simulink model "adc16_dbf_4fft"  (R2013a)
settings: Solver=ode45  StartTime=0.0  StopTime=2050  RelTol=1e-3
undefined symbols (not defined in the file): pfb_coeff_gen_calc
libraries: xbsIndex_r4 x1713, casper_library_misc x294, casper_library_delays x48, casper_library_pfbs x16, simulink x16, xps_library x1
(part 4 of 21)

== system adc16_dbf_4fft/sync_gen ==
  Constant : Constant
  Constant1 : Constant  Value=0
  Constant2 : Constant  Value=0
  Counter3 : xbsIndex_r4/Counter  cnt_type=Free Running  cnt_to=Inf  operation=Up  start_count=0  cnt_by_val=1  arith_type=Unsigned  n_bits=32  bin_pt=0  load_pin=off  rst=on  en=off  explicit_period=off  period=1  dbl_ovrd=off  use_behavioral_HDL=on  implementation=Fabric  use_rpm=on  block_type=counter
      settings: xl_area=[0, 0, 0, 0, 0, 0, 0]
  Logical : xbsIndex_r4/Logical  logical_function=OR  inputs=2  en=off  latency=0  precision=Full  arith_type=Unsigned  n_bits=8  bin_pt=2  align_bp=on  dbl_ovrd=off  block_type=logical
      settings: xl_area=[0, 0, 0, 0, 0, 0, 0]
  Logical1 : xbsIndex_r4/Logical  logical_function=OR  inputs=2  en=off  latency=0  precision=Full  arith_type=Unsigned  n_bits=8  bin_pt=2  align_bp=on  dbl_ovrd=off  block_type=logical
      settings: xl_area=[0, 0, 0, 0, 0, 0, 0]
  Mux : xbsIndex_r4/Mux  inputs=2  en=off  latency=0  precision=Full  arith_type=Unsigned  n_bits=16  bin_pt=14  quantization=Truncate  overflow=Wrap  dbl_ovrd=off  block_type=mux
  Relational : xbsIndex_r4/Relational  mode=a=b  en=off  latency=1  dbl_ovrd=off  block_type=relational
      settings: xl_area=[0, 0, 0, 0, 0, 0, 0]  block_version=10.1.3
  Slice1 : xbsIndex_r4/Slice  nbits=1  boolean_output=on  mode=Lower Bit Location + Width  bit1=0  base1=MSB of Input  bit0=0  base0=LSB of Input  dbl_ovrd=off  block_type=slice
      settings: infoedit="Extracts a given range of bits from each input sample and presents it at the output.  The output type is ordinarily unsigned with binary point at zero, but can be Boolean when the slice is one bit wide.<P><P>Hardware notes: In hardware this block costs nothing."  block_version=10.1.3
  Slice2 : xbsIndex_r4/Slice  nbits=1  boolean_output=on  mode=Lower Bit Location + Width  bit1=0  base1=MSB of Input  bit0=0  base0=LSB of Input  dbl_ovrd=off  block_type=slice
      settings: infoedit="Extracts a given range of bits from each input sample and presents it at the output.  The output type is ordinarily unsigned with binary point at zero, but can be Boolean when the slice is one bit wide.<P><P>Hardware notes: In hardware this block costs nothing."  block_version=10.1.3
  posedge1 : casper_library_misc/edge_detect  edge=Rising  polarity=Active High  x_in=[0 0.08 0.08 0.16 0.16 0.24 0.24 0.32 0.32 0.4]  y_in="[-1 -1  1  1  1  1  1  1  1  1]"  x_out=[0.6 0.68 0.68 0.76 0.76 0.84 0.84 0.92 0.92 1]  y_out="[-1 -1  1  1 -1 -1 -1 -1 -1 -1]"
  posedge3 : casper_library_misc/edge_detect  edge=Rising  polarity=Active High  x_in=[0 0.08 0.08 0.16 0.16 0.24 0.24 0.32 0.32 0.4]  y_in="[-1 -1  1  1  1  1  1  1  1  1]"  x_out=[0.6 0.68 0.68 0.76 0.76 0.84 0.84 0.92 0.92 1]  y_out="[-1 -1  1  1 -1 -1 -1 -1 -1 -1]"
  sync : Subsystem  Tag=xps:sw_reg  AncestorBlock=xps_library/software_register  mask(swreg){mode=one value, io_dir=From Processor, io_delay=0, sample_period=1, names=reg, bitwidths=32, arith_types=0, bin_pts=0, sim_port=on, show_format=off}
      mask prompts: io_dir "I/O direction"; io_delay "I/O delay"; sample_period "Sample period"; names "Name:"; bitwidths "Bitwidth:"; arith_types "Type (ufix=0, fix=1, bool=2):"; bin_pts "Binary pt:"; sim_port "Provide sim input/output?"; show_format "Print format string?"
      mask init:
      | swreg_init(gcb)
      settings: AttributesFormatString=1input
      mask TypeOptions mode: one value | fields of equal size | fields of arbitrary size
      mask Callback mode: swreg_cb(gcb);
      mask TypeOptions io_dir: To Processor | From Processor
      mask Callback io_dir:
      | mask_enables = get_param(gcb, 'MaskEnables');
      | mask_names = get_param(gcb, 'MaskNames');
      | if strcmp(get_param(gcb, 'io_dir'), 'To Processor'),
      |     mask_enables{ismember(mask_names, 'sample_period')} = 'off';
      | else
      |     mask_enables{ismember(mask_names, 'sample_period')} = 'on';
      | end
      | set_param(gcb, 'MaskEnables', mask_enables);
      mask Callback bitwidths:
      | swreg_maskcheck(gcb);
      | % blk = gcb;
      | % mode = get_param(blk, 'mode');
      | % current_widths = eval(get_param(blk, 'bitwidths'));
      | % if (strcmp(mode, 'one value') || strcmp(mode, 'fields of equal size')) && (length(current_widths) > 1),
      | %     error('Only one width may be specified for this mode.');
      | % elseif strcmp(mode, 'fields of arbitrary size')
      | %     current_names = textscan(strtrim(strrep(strrep(get_param(blk, 'names'), ']', ''), '[', '')), '%s');
      | %     current_names = current_names{1};
      | %     numios = length(current_names);
      | %     if length(current_widths) ~= numios,
      | %         error('%d field names specified, but %d widths?', numios, length(current_widths));
      | %     end
      | % end
      | % total_width = 0;
      | % for ctr = 1 : length(current_widths),
      | %     total_width = total_width + current_widths(ctr);
      | % end
      | % if total_width > 32,
      | %     error('Total width must be 32 or less, set to %d.', total_width);
      | % end
      mask Callback arith_types:
      | [numios, ~, ~, ~, current_types] = swreg_maskcheck(gcb);
      | % blk = gcb;
      | % mode = get_param(blk, 'mode');
      | % current_types = eval(get_param(blk, 'arith_types'));
      | % numios = length(current_types);
      | % if (strcmp(mode, 'one value') || strcmp(mode, 'fields of equal size')) && (length(current_types) > 1),
      | %     error('Only one type may be specified for this mode.');
      | % elseif strcmp(mode, 'fields of arbitrary size')
      | %     current_names = textscan(strtrim(strrep(strrep(get_param(blk, 'names'), ']', ''), '[', '')), '%s');
      | %     current_names = current_names{1};
      | %     numios = length(current_names);
      | %     if length(current_types) ~= numios,
      | %         error('%d field names specified, but %d types?', numios, length(current_types));
      | %     end
      | % end
      | problem = 0;
      | for ctr = 1 : numios,
      |     t = current_types(ctr);
      |     if (t < 0) || (t > 2),
      |         problem = t;
      |         ctr = numios + 1;
      |     end
      | end
      | if problem ~= 0,
      |     error('Type cannot be %i, must be 0, 1 or 2.', problem);
      | end
      mask Callback bin_pts:
      | swreg_maskcheck(gcb);
      | % blk = gcb;
      | % mode = get_param(blk, 'mode');
      | % current_bins = eval(get_param(blk, 'bin_pts'));
      | % if (strcmp(mode, 'one value') || strcmp(mode, 'fields of equal size')) && (length(current_bins) > 1),
      | %     error('Only one binary pt may be specified for this mode.');
      | % elseif strcmp(mode, 'fields of arbitrary size')
      | %     current_names = textscan(strtrim(strrep(strrep(get_param(blk, 'names'), ']', ''), '[', '')), '%s');
      | %     current_names = current_names{1};
      | %     numios = length(current_names);
      | %     if length(current_bins) ~= numios,
      | %         error('%d field names specified, but %d binary pts?', numios, length(current_bins));
      | %     end
      | % end
  sync_period_const : xbsIndex_r4/Constant  const=1022  gui_display_data_type=Fixed-point  arith_type=Signed (2's comp)  n_bits=32  bin_pt=0  preci_type=Single  exp_width=8  frac_width=24  explicit_period=off  period=1  equ=P=C  opselect=C  inp2=PCIN>>17  opr=+  inp1=P  carry=CIN  dbl_ovrd=off  block_type=constant
      settings: block_version=10.1.1
  sync_period_sel : Subsystem  Tag=xps:sw_reg  AncestorBlock=xps_library/software_register  mask(swreg){mode=one value, io_dir=From Processor, io_delay=0, sample_period=1, names=reg, bitwidths=32, arith_types=0, bin_pts=0, sim_port=on, show_format=off}
      mask prompts: io_dir "I/O direction"; io_delay "I/O delay"; sample_period "Sample period"; names "Name:"; bitwidths "Bitwidth:"; arith_types "Type (ufix=0, fix=1, bool=2):"; bin_pts "Binary pt:"; sim_port "Provide sim input/output?"; show_format "Print format string?"
      mask init:
      | swreg_init(gcb)
      settings: AttributesFormatString=1input
      mask TypeOptions mode: one value | fields of equal size | fields of arbitrary size
      mask Callback mode: swreg_cb(gcb);
      mask TypeOptions io_dir: To Processor | From Processor
      mask Callback io_dir:
      | mask_enables = get_param(gcb, 'MaskEnables');
      | mask_names = get_param(gcb, 'MaskNames');
      | if strcmp(get_param(gcb, 'io_dir'), 'To Processor'),
      |     mask_enables{ismember(mask_names, 'sample_period')} = 'off';
      | else
      |     mask_enables{ismember(mask_names, 'sample_period')} = 'on';
      | end
      | set_param(gcb, 'MaskEnables', mask_enables);
      mask Callback bitwidths:
      | swreg_maskcheck(gcb);
      | % blk = gcb;
      | % mode = get_param(blk, 'mode');
      | % current_widths = eval(get_param(blk, 'bitwidths'));
      | % if (strcmp(mode, 'one value') || strcmp(mode, 'fields of equal size')) && (length(current_widths) > 1),
      | %     error('Only one width may be specified for this mode.');
      | % elseif strcmp(mode, 'fields of arbitrary size')
      | %     current_names = textscan(strtrim(strrep(strrep(get_param(blk, 'names'), ']', ''), '[', '')), '%s');
      | %     current_names = current_names{1};
      | %     numios = length(current_names);
      | %     if length(current_widths) ~= numios,
      | %         error('%d field names specified, but %d widths?', numios, length(current_widths));
      | %     end
      | % end
      | % total_width = 0;
      | % for ctr = 1 : length(current_widths),
      | %     total_width = total_width + current_widths(ctr);
      | % end
      | % if total_width > 32,
      | %     error('Total width must be 32 or less, set to %d.', total_width);
      | % end
      mask Callback arith_types:
      | [numios, ~, ~, ~, current_types] = swreg_maskcheck(gcb);
      | % blk = gcb;
      | % mode = get_param(blk, 'mode');
      | % current_types = eval(get_param(blk, 'arith_types'));
      | % numios = length(current_types);
      | % if (strcmp(mode, 'one value') || strcmp(mode, 'fields of equal size')) && (length(current_types) > 1),
      | %     error('Only one type may be specified for this mode.');
      | % elseif strcmp(mode, 'fields of arbitrary size')
      | %     current_names = textscan(strtrim(strrep(strrep(get_param(blk, 'names'), ']', ''), '[', '')), '%s');
      | %     current_names = current_names{1};
      | %     numios = length(current_names);
      | %     if length(current_types) ~= numios,
      | %         error('%d field names specified, but %d types?', numios, length(current_types));
      | %     end
      | % end
      | problem = 0;
      | for ctr = 1 : numios,
      |     t = current_types(ctr);
      |     if (t < 0) || (t > 2),
      |         problem = t;
      |         ctr = numios + 1;
      |     end
      | end
      | if problem ~= 0,
      |     error('Type cannot be %i, must be 0, 1 or 2.', problem);
      | end
      mask Callback bin_pts:
      | swreg_maskcheck(gcb);
      | % blk = gcb;
      | % mode = get_param(blk, 'mode');
      | % current_bins = eval(get_param(blk, 'bin_pts'));
      | % if (strcmp(mode, 'one value') || strcmp(mode, 'fields of equal size')) && (length(current_bins) > 1),
      | %     error('Only one binary pt may be specified for this mode.');
      | % elseif strcmp(mode, 'fields of arbitrary size')
      | %     current_names = textscan(strtrim(strrep(strrep(get_param(blk, 'names'), ']', ''), '[', '')), '%s');
      | %     current_names = current_names{1};
      | %     numios = length(current_names);
      | %     if length(current_bins) ~= numios,
      | %         error('%d field names specified, but %d binary pts?', numios, length(current_bins));
      | %     end
      | % end
  sync_period_var : Subsystem  Tag=xps:sw_reg  AncestorBlock=xps_library/software_register  mask(swreg){mode=one value, io_dir=From Processor, io_delay=0, sample_period=1, names=reg, bitwidths=32, arith_types=0, bin_pts=0, sim_port=on, show_format=off}
      mask prompts: io_dir "I/O direction"; io_delay "I/O delay"; sample_period "Sample period"; names "Name:"; bitwidths "Bitwidth:"; arith_types "Type (ufix=0, fix=1, bool=2):"; bin_pts "Binary pt:"; sim_port "Provide sim input/output?"; show_format "Print format string?"
      mask init:
      | swreg_init(gcb)
      settings: AttributesFormatString=1input
      mask TypeOptions mode: one value | fields of equal size | fields of arbitrary size
      mask Callback mode: swreg_cb(gcb);
      mask TypeOptions io_dir: To Processor | From Processor
      mask Callback io_dir:
      | mask_enables = get_param(gcb, 'MaskEnables');
      | mask_names = get_param(gcb, 'MaskNames');
      | if strcmp(get_param(gcb, 'io_dir'), 'To Processor'),
      |     mask_enables{ismember(mask_names, 'sample_period')} = 'off';
      | else
      |     mask_enables{ismember(mask_names, 'sample_period')} = 'on';
      | end
      | set_param(gcb, 'MaskEnables', mask_enables);
      mask Callback bitwidths:
      | swreg_maskcheck(gcb);
      | % blk = gcb;
      | % mode = get_param(blk, 'mode');
      | % current_widths = eval(get_param(blk, 'bitwidths'));
      | % if (strcmp(mode, 'one value') || strcmp(mode, 'fields of equal size')) && (length(current_widths) > 1),
      | %     error('Only one width may be specified for this mode.');
      | % elseif strcmp(mode, 'fields of arbitrary size')
      | %     current_names = textscan(strtrim(strrep(strrep(get_param(blk, 'names'), ']', ''), '[', '')), '%s');
      | %     current_names = current_names{1};
      | %     numios = length(current_names);
      | %     if length(current_widths) ~= numios,
      | %         error('%d field names specified, but %d widths?', numios, length(current_widths));
      | %     end
      | % end
      | % total_width = 0;
      | % for ctr = 1 : length(current_widths),
      | %     total_width = total_width + current_widths(ctr);
      | % end
      | % if total_width > 32,
      | %     error('Total width must be 32 or less, set to %d.', total_width);
      | % end
      mask Callback arith_types:
      | [numios, ~, ~, ~, current_types] = swreg_maskcheck(gcb);
      | % blk = gcb;
      | % mode = get_param(blk, 'mode');
      | % current_types = eval(get_param(blk, 'arith_types'));
      | % numios = length(current_types);
      | % if (strcmp(mode, 'one value') || strcmp(mode, 'fields of equal size')) && (length(current_types) > 1),
      | %     error('Only one type may be specified for this mode.');
      | % elseif strcmp(mode, 'fields of arbitrary size')
      | %     current_names = textscan(strtrim(strrep(strrep(get_param(blk, 'names'), ']', ''), '[', '')), '%s');
      | %     current_names = current_names{1};
      | %     numios = length(current_names);
      | %     if length(current_types) ~= numios,
      | %         error('%d field names specified, but %d types?', numios, length(current_types));
      | %     end
      | % end
      | problem = 0;
      | for ctr = 1 : numios,
      |     t = current_types(ctr);
      |     if (t < 0) || (t > 2),
      |         problem = t;
      |         ctr = numios + 1;
      |     end
      | end
      | if problem ~= 0,
      |     error('Type cannot be %i, must be 0, 1 or 2.', problem);
      | end
      mask Callback bin_pts:
      | swreg_maskcheck(gcb);
      | % blk = gcb;
      | % mode = get_param(blk, 'mode');
      | % current_bins = eval(get_param(blk, 'bin_pts'));
      | % if (strcmp(mode, 'one value') || strcmp(mode, 'fields of equal size')) && (length(current_bins) > 1),
      | %     error('Only one binary pt may be specified for this mode.');
      | % elseif strcmp(mode, 'fields of arbitrary size')
      | %     current_names = textscan(strtrim(strrep(strrep(get_param(blk, 'names'), ']', ''), '[', '')), '%s');
      | %     current_names = current_names{1};
      | %     numios = length(current_names);
      | %     if length(current_bins) ~= numios,
      | %         error('%d field names specified, but %d binary pts?', numios, length(current_bins));
      | %     end
      | % end
  sync_out : Outport
  wires:
  Constant2/1 -> sync_period_var/1(sim_1)
  sync_period_var/1(in_reg) -> Mux/3
  sync_period_const/1 -> Mux/2
  Slice1/1 -> Mux/1
  sync_period_sel/1(in_reg) -> Slice1/1
  Constant1/1 -> sync_period_sel/1(sim_1)
  Mux/1 -> Relational/1
  posedge1/1 -> sync_out/1
  Logical/1 -> posedge1/1
  Relational/1 -> Logical1/1, Logical/1
  Counter3/1 -> Relational/2
  Logical1/1 -> Counter3/1
  Slice2/1 -> Logical/2, Logical1/2
  posedge3/1 -> Slice2/1
  sync/1(in_reg) -> posedge3/1
  Constant/1 -> sync/1(sim_1)

== system adc16_dbf_4fft/4fft/mult_j ==
  a+jb : Inport
  Negate : xbsIndex_r4/Negate  precision=User Defined  arith_type="Signed  (2's comp)"  n_bits=18  bin_pt=17  quantization=Truncate  overflow=Wrap  en=off  latency=0  dbl_ovrd=off  block_type=negate
  c_to_ri : casper_library_misc/c_to_ri  n_bits=18  bin_pt=17
  ri_to_c : casper_library_misc/ri_to_c
  ja-b : Outport
  wires:
  a+jb/1 -> c_to_ri/1
  ri_to_c/1 -> ja-b/1
  c_to_ri/2 -> Negate/1
  c_to_ri/1 -> ri_to_c/2
  Negate/1 -> ri_to_c/1

== system adc16_dbf_4fft/4fft/mult_jjj ==
  a+jb : Inport
  Negate : xbsIndex_r4/Negate  precision=User Defined  arith_type="Signed  (2's comp)"  n_bits=18  bin_pt=17  quantization=Truncate  overflow=Wrap  en=off  latency=0  dbl_ovrd=off  block_type=negate
  c_to_ri : casper_library_misc/c_to_ri  n_bits=18  bin_pt=17
  ri_to_c : casper_library_misc/ri_to_c
  b-ja : Outport
  wires:
  ri_to_c/1 -> b-ja/1
  a+jb/1 -> c_to_ri/1
  c_to_ri/2 -> ri_to_c/1
  c_to_ri/1 -> Negate/1
  Negate/1 -> ri_to_c/2

== system adc16_dbf_4fft/4fft/pipeline ==
  d : Inport
  Register{0..3} (4 alike) : xbsIndex_r4/Register  init=0  rst=off  en=off  dbl_ovrd=off  block_type=register
      Register0 settings: block_version=11.4
      Register1 settings: block_version=11.4
  q : Outport
  wires:
  Register0/1 -> Register1/1
  Register1/1 -> Register2/1
  Register2/1 -> Register3/1
  d/1 -> Register0/1
  Register3/1 -> q/1

== system adc16_dbf_4fft/4fft/pipeline1 ==
  d : Inport
  Register{0..3} (4 alike) : xbsIndex_r4/Register  init=0  rst=off  en=off  dbl_ovrd=off  block_type=register
      Register0 settings: block_version=11.4
      Register1 settings: block_version=11.4
  q : Outport
  wires:
  Register0/1 -> Register1/1
  Register1/1 -> Register2/1
  Register2/1 -> Register3/1
  d/1 -> Register0/1
  Register3/1 -> q/1

== system adc16_dbf_4fft/4fft/real2complex ==
  r : Inport
  c_to_ri : casper_library_misc/c_to_ri  n_bits=18  bin_pt=17
  ri_to_c : casper_library_misc/ri_to_c
  c : Outport
  wires:
  c_to_ri/2 -> ri_to_c/2
  r/1 -> c_to_ri/1
  c_to_ri/1 -> ri_to_c/1
  ri_to_c/1 -> c/1

== system adc16_dbf_4fft/4fft/real2complex1 ==
  r : Inport
  c_to_ri : casper_library_misc/c_to_ri  n_bits=18  bin_pt=17
  ri_to_c : casper_library_misc/ri_to_c
  c : Outport
  wires:
  ri_to_c/1 -> c/1
  c_to_ri/1 -> ri_to_c/1
  r/1 -> c_to_ri/1
  c_to_ri/2 -> ri_to_c/2

== system adc16_dbf_4fft/4fft/real2complex2 ==
  r : Inport
  c_to_ri : casper_library_misc/c_to_ri  n_bits=18  bin_pt=17
  ri_to_c : casper_library_misc/ri_to_c
  c : Outport
  wires:
  c_to_ri/2 -> ri_to_c/2
  r/1 -> c_to_ri/1
  c_to_ri/1 -> ri_to_c/1
  ri_to_c/1 -> c/1

== system adc16_dbf_4fft/4fft/real2complex3 ==
  r : Inport
  c_to_ri : casper_library_misc/c_to_ri  n_bits=18  bin_pt=17
  ri_to_c : casper_library_misc/ri_to_c
  c : Outport
  wires:
  ri_to_c/1 -> c/1
  c_to_ri/1 -> ri_to_c/1
  r/1 -> c_to_ri/1
  c_to_ri/2 -> ri_to_c/2

== system adc16_dbf_4fft/4fft1/mult_j ==
  a+jb : Inport
  Negate : xbsIndex_r4/Negate  precision=User Defined  arith_type="Signed  (2's comp)"  n_bits=18  bin_pt=17  quantization=Truncate  overflow=Wrap  en=off  latency=0  dbl_ovrd=off  block_type=negate
  c_to_ri : casper_library_misc/c_to_ri  n_bits=18  bin_pt=17
  ri_to_c : casper_library_misc/ri_to_c
  ja-b : Outport
  wires:
  Negate/1 -> ri_to_c/1
  c_to_ri/1 -> ri_to_c/2
  c_to_ri/2 -> Negate/1
  ri_to_c/1 -> ja-b/1
  a+jb/1 -> c_to_ri/1

== system adc16_dbf_4fft/4fft1/mult_jjj ==
  a+jb : Inport
  Negate : xbsIndex_r4/Negate  precision=User Defined  arith_type="Signed  (2's comp)"  n_bits=18  bin_pt=17  quantization=Truncate  overflow=Wrap  en=off  latency=0  dbl_ovrd=off  block_type=negate
  c_to_ri : casper_library_misc/c_to_ri  n_bits=18  bin_pt=17
  ri_to_c : casper_library_misc/ri_to_c
  b-ja : Outport
  wires:
  Negate/1 -> ri_to_c/2
  c_to_ri/1 -> Negate/1
  c_to_ri/2 -> ri_to_c/1
  a+jb/1 -> c_to_ri/1
  ri_to_c/1 -> b-ja/1

== system adc16_dbf_4fft/4fft1/pipeline ==
  d : Inport
  Register{0..3} (4 alike) : xbsIndex_r4/Register  init=0  rst=off  en=off  dbl_ovrd=off  block_type=register
      Register0 settings: block_version=11.4
      Register1 settings: block_version=11.4
  q : Outport
  wires:
  Register3/1 -> q/1
  d/1 -> Register0/1
  Register2/1 -> Register3/1
  Register1/1 -> Register2/1
  Register0/1 -> Register1/1

== system adc16_dbf_4fft/4fft1/pipeline1 ==
  d : Inport
  Register{0..3} (4 alike) : xbsIndex_r4/Register  init=0  rst=off  en=off  dbl_ovrd=off  block_type=register
      Register0 settings: block_version=11.4
      Register1 settings: block_version=11.4
  q : Outport
  wires:
  Register3/1 -> q/1
  d/1 -> Register0/1
  Register2/1 -> Register3/1
  Register1/1 -> Register2/1
  Register0/1 -> Register1/1

== system adc16_dbf_4fft/4fft1/real2complex ==
  r : Inport
  c_to_ri : casper_library_misc/c_to_ri  n_bits=18  bin_pt=17
  ri_to_c : casper_library_misc/ri_to_c
  c : Outport
  wires:
  ri_to_c/1 -> c/1
  c_to_ri/1 -> ri_to_c/1
  r/1 -> c_to_ri/1
  c_to_ri/2 -> ri_to_c/2

== system adc16_dbf_4fft/4fft1/real2complex1 ==
  r : Inport
  c_to_ri : casper_library_misc/c_to_ri  n_bits=18  bin_pt=17
  ri_to_c : casper_library_misc/ri_to_c
  c : Outport
  wires:
  c_to_ri/2 -> ri_to_c/2
  r/1 -> c_to_ri/1
  c_to_ri/1 -> ri_to_c/1
  ri_to_c/1 -> c/1

== system adc16_dbf_4fft/4fft1/real2complex2 ==
  r : Inport
  c_to_ri : casper_library_misc/c_to_ri  n_bits=18  bin_pt=17
  ri_to_c : casper_library_misc/ri_to_c
  c : Outport
  wires:
  ri_to_c/1 -> c/1
  c_to_ri/1 -> ri_to_c/1
  r/1 -> c_to_ri/1
  c_to_ri/2 -> ri_to_c/2

== system adc16_dbf_4fft/4fft1/real2complex3 ==
  r : Inport
  c_to_ri : casper_library_misc/c_to_ri  n_bits=18  bin_pt=17
  ri_to_c : casper_library_misc/ri_to_c
  c : Outport
  wires:
  c_to_ri/2 -> ri_to_c/2
  r/1 -> c_to_ri/1
  c_to_ri/1 -> ri_to_c/1
  ri_to_c/1 -> c/1

== system adc16_dbf_4fft/4fft2/mult_j ==
  a+jb : Inport
  Negate : xbsIndex_r4/Negate  precision=User Defined  arith_type="Signed  (2's comp)"  n_bits=18  bin_pt=17  quantization=Truncate  overflow=Wrap  en=off  latency=0  dbl_ovrd=off  block_type=negate
  c_to_ri : casper_library_misc/c_to_ri  n_bits=18  bin_pt=17
  ri_to_c : casper_library_misc/ri_to_c
  ja-b : Outport
  wires:
  a+jb/1 -> c_to_ri/1
  ri_to_c/1 -> ja-b/1
  c_to_ri/2 -> Negate/1
  c_to_ri/1 -> ri_to_c/2
  Negate/1 -> ri_to_c/1

== system adc16_dbf_4fft/4fft2/mult_jjj ==
  a+jb : Inport
  Negate : xbsIndex_r4/Negate  precision=User Defined  arith_type="Signed  (2's comp)"  n_bits=18  bin_pt=17  quantization=Truncate  overflow=Wrap  en=off  latency=0  dbl_ovrd=off  block_type=negate
  c_to_ri : casper_library_misc/c_to_ri  n_bits=18  bin_pt=17
  ri_to_c : casper_library_misc/ri_to_c
  b-ja : Outport
  wires:
  ri_to_c/1 -> b-ja/1
  a+jb/1 -> c_to_ri/1
  c_to_ri/2 -> ri_to_c/1
  c_to_ri/1 -> Negate/1
  Negate/1 -> ri_to_c/2

== system adc16_dbf_4fft/4fft2/pipeline ==
  d : Inport
  Register{0..3} (4 alike) : xbsIndex_r4/Register  init=0  rst=off  en=off  dbl_ovrd=off  block_type=register
      Register0 settings: block_version=11.4
      Register1 settings: block_version=11.4
  q : Outport
  wires:
  Register0/1 -> Register1/1
  Register1/1 -> Register2/1
  Register2/1 -> Register3/1
  d/1 -> Register0/1
  Register3/1 -> q/1

== system adc16_dbf_4fft/4fft2/pipeline1 ==
  d : Inport
  Register{0..3} (4 alike) : xbsIndex_r4/Register  init=0  rst=off  en=off  dbl_ovrd=off  block_type=register
      Register0 settings: block_version=11.4
      Register1 settings: block_version=11.4
  q : Outport
  wires:
  Register0/1 -> Register1/1
  Register1/1 -> Register2/1
  Register2/1 -> Register3/1
  d/1 -> Register0/1
  Register3/1 -> q/1

== system adc16_dbf_4fft/4fft2/real2complex ==
  r : Inport
  c_to_ri : casper_library_misc/c_to_ri  n_bits=18  bin_pt=17
  ri_to_c : casper_library_misc/ri_to_c
  c : Outport
  wires:
  c_to_ri/2 -> ri_to_c/2
  r/1 -> c_to_ri/1
  c_to_ri/1 -> ri_to_c/1
  ri_to_c/1 -> c/1

== system adc16_dbf_4fft/4fft2/real2complex1 ==
  r : Inport
  c_to_ri : casper_library_misc/c_to_ri  n_bits=18  bin_pt=17
  ri_to_c : casper_library_misc/ri_to_c
  c : Outport
  wires:
  ri_to_c/1 -> c/1
  c_to_ri/1 -> ri_to_c/1
  r/1 -> c_to_ri/1
  c_to_ri/2 -> ri_to_c/2

== system adc16_dbf_4fft/4fft2/real2complex2 ==
  r : Inport
  c_to_ri : casper_library_misc/c_to_ri  n_bits=18  bin_pt=17
  ri_to_c : casper_library_misc/ri_to_c
  c : Outport
  wires:
  c_to_ri/2 -> ri_to_c/2
  r/1 -> c_to_ri/1
  c_to_ri/1 -> ri_to_c/1
  ri_to_c/1 -> c/1

== system adc16_dbf_4fft/4fft2/real2complex3 ==
  r : Inport
  c_to_ri : casper_library_misc/c_to_ri  n_bits=18  bin_pt=17
  ri_to_c : casper_library_misc/ri_to_c
  c : Outport
  wires:
  ri_to_c/1 -> c/1
  c_to_ri/1 -> ri_to_c/1
  r/1 -> c_to_ri/1
  c_to_ri/2 -> ri_to_c/2

== system adc16_dbf_4fft/4fft3/mult_j ==
  a+jb : Inport
  Negate : xbsIndex_r4/Negate  precision=User Defined  arith_type="Signed  (2's comp)"  n_bits=18  bin_pt=17  quantization=Truncate  overflow=Wrap  en=off  latency=0  dbl_ovrd=off  block_type=negate
  c_to_ri : casper_library_misc/c_to_ri  n_bits=18  bin_pt=17
  ri_to_c : casper_library_misc/ri_to_c
  ja-b : Outport
  wires:
  Negate/1 -> ri_to_c/1
  c_to_ri/1 -> ri_to_c/2
  c_to_ri/2 -> Negate/1
  ri_to_c/1 -> ja-b/1
  a+jb/1 -> c_to_ri/1

== system adc16_dbf_4fft/4fft3/mult_jjj ==
  a+jb : Inport
  Negate : xbsIndex_r4/Negate  precision=User Defined  arith_type="Signed  (2's comp)"  n_bits=18  bin_pt=17  quantization=Truncate  overflow=Wrap  en=off  latency=0  dbl_ovrd=off  block_type=negate
  c_to_ri : casper_library_misc/c_to_ri  n_bits=18  bin_pt=17
  ri_to_c : casper_library_misc/ri_to_c
  b-ja : Outport
  wires:
  Negate/1 -> ri_to_c/2
  c_to_ri/1 -> Negate/1
  c_to_ri/2 -> ri_to_c/1
  a+jb/1 -> c_to_ri/1
  ri_to_c/1 -> b-ja/1

== system adc16_dbf_4fft/4fft3/pipeline ==
  d : Inport
  Register{0..3} (4 alike) : xbsIndex_r4/Register  init=0  rst=off  en=off  dbl_ovrd=off  block_type=register
      Register0 settings: block_version=11.4
      Register1 settings: block_version=11.4
  q : Outport
  wires:
  Register3/1 -> q/1
  d/1 -> Register0/1
  Register2/1 -> Register3/1
  Register1/1 -> Register2/1
  Register0/1 -> Register1/1

== system adc16_dbf_4fft/4fft3/pipeline1 ==
  d : Inport
  Register{0..3} (4 alike) : xbsIndex_r4/Register  init=0  rst=off  en=off  dbl_ovrd=off  block_type=register
      Register0 settings: block_version=11.4
      Register1 settings: block_version=11.4
  q : Outport
  wires:
  Register3/1 -> q/1
  d/1 -> Register0/1
  Register2/1 -> Register3/1
  Register1/1 -> Register2/1
  Register0/1 -> Register1/1

== system adc16_dbf_4fft/4fft3/real2complex ==
  r : Inport
  c_to_ri : casper_library_misc/c_to_ri  n_bits=18  bin_pt=17
  ri_to_c : casper_library_misc/ri_to_c
  c : Outport
  wires:
  ri_to_c/1 -> c/1
  c_to_ri/1 -> ri_to_c/1
  r/1 -> c_to_ri/1
  c_to_ri/2 -> ri_to_c/2

== system adc16_dbf_4fft/4fft3/real2complex1 ==
  r : Inport
  c_to_ri : casper_library_misc/c_to_ri  n_bits=18  bin_pt=17
  ri_to_c : casper_library_misc/ri_to_c
  c : Outport
  wires:
  c_to_ri/2 -> ri_to_c/2
  r/1 -> c_to_ri/1
  c_to_ri/1 -> ri_to_c/1
  ri_to_c/1 -> c/1

== system adc16_dbf_4fft/4fft3/real2complex2 ==
  r : Inport
  c_to_ri : casper_library_misc/c_to_ri  n_bits=18  bin_pt=17
  ri_to_c : casper_library_misc/ri_to_c
  c : Outport
  wires:
  ri_to_c/1 -> c/1
  c_to_ri/1 -> ri_to_c/1
  r/1 -> c_to_ri/1
  c_to_ri/2 -> ri_to_c/2

== system adc16_dbf_4fft/4fft3/real2complex3 ==
  r : Inport
  c_to_ri : casper_library_misc/c_to_ri  n_bits=18  bin_pt=17
  ri_to_c : casper_library_misc/ri_to_c
  c : Outport
  wires:
  c_to_ri/2 -> ri_to_c/2
  r/1 -> c_to_ri/1
  c_to_ri/1 -> ri_to_c/1
  ri_to_c/1 -> c/1

== system adc16_dbf_4fft/4fft4/mult_j ==
  a+jb : Inport
  Negate : xbsIndex_r4/Negate  precision=User Defined  arith_type="Signed  (2's comp)"  n_bits=18  bin_pt=17  quantization=Truncate  overflow=Wrap  en=off  latency=0  dbl_ovrd=off  block_type=negate
  c_to_ri : casper_library_misc/c_to_ri  n_bits=18  bin_pt=17
  ri_to_c : casper_library_misc/ri_to_c
  ja-b : Outport
  wires:
  a+jb/1 -> c_to_ri/1
  ri_to_c/1 -> ja-b/1
  c_to_ri/2 -> Negate/1
  c_to_ri/1 -> ri_to_c/2
  Negate/1 -> ri_to_c/1

== system adc16_dbf_4fft/4fft4/mult_jjj ==
  a+jb : Inport
  Negate : xbsIndex_r4/Negate  precision=User Defined  arith_type="Signed  (2's comp)"  n_bits=18  bin_pt=17  quantization=Truncate  overflow=Wrap  en=off  latency=0  dbl_ovrd=off  block_type=negate
  c_to_ri : casper_library_misc/c_to_ri  n_bits=18  bin_pt=17
  ri_to_c : casper_library_misc/ri_to_c
  b-ja : Outport
  wires:
  ri_to_c/1 -> b-ja/1
  a+jb/1 -> c_to_ri/1
  c_to_ri/2 -> ri_to_c/1
  c_to_ri/1 -> Negate/1
  Negate/1 -> ri_to_c/2

== system adc16_dbf_4fft/4fft4/pipeline ==
  d : Inport
  Register{0..3} (4 alike) : xbsIndex_r4/Register  init=0  rst=off  en=off  dbl_ovrd=off  block_type=register
      Register0 settings: block_version=11.4
      Register1 settings: block_version=11.4
  q : Outport
  wires:
  Register0/1 -> Register1/1
  Register1/1 -> Register2/1
  Register2/1 -> Register3/1
  d/1 -> Register0/1
  Register3/1 -> q/1

== system adc16_dbf_4fft/4fft4/pipeline1 ==
  d : Inport
  Register{0..3} (4 alike) : xbsIndex_r4/Register  init=0  rst=off  en=off  dbl_ovrd=off  block_type=register
      Register0 settings: block_version=11.4
      Register1 settings: block_version=11.4
  q : Outport
  wires:
  Register0/1 -> Register1/1
  Register1/1 -> Register2/1
  Register2/1 -> Register3/1
  d/1 -> Register0/1
  Register3/1 -> q/1

== system adc16_dbf_4fft/4fft4/real2complex ==
  r : Inport
  c_to_ri : casper_library_misc/c_to_ri  n_bits=18  bin_pt=17
  ri_to_c : casper_library_misc/ri_to_c
  c : Outport
  wires:
  c_to_ri/2 -> ri_to_c/2
  r/1 -> c_to_ri/1
  c_to_ri/1 -> ri_to_c/1
  ri_to_c/1 -> c/1

== system adc16_dbf_4fft/4fft4/real2complex1 ==
  r : Inport
  c_to_ri : casper_library_misc/c_to_ri  n_bits=18  bin_pt=17
  ri_to_c : casper_library_misc/ri_to_c
  c : Outport
  wires:
  ri_to_c/1 -> c/1
  c_to_ri/1 -> ri_to_c/1
  r/1 -> c_to_ri/1
  c_to_ri/2 -> ri_to_c/2

== system adc16_dbf_4fft/4fft4/real2complex2 ==
  r : Inport
  c_to_ri : casper_library_misc/c_to_ri  n_bits=18  bin_pt=17
  ri_to_c : casper_library_misc/ri_to_c
  c : Outport
  wires:
  c_to_ri/2 -> ri_to_c/2
  r/1 -> c_to_ri/1
  c_to_ri/1 -> ri_to_c/1
  ri_to_c/1 -> c/1

== system adc16_dbf_4fft/4fft4/real2complex3 ==
  r : Inport
  c_to_ri : casper_library_misc/c_to_ri  n_bits=18  bin_pt=17
  ri_to_c : casper_library_misc/ri_to_c
  c : Outport
  wires:
  ri_to_c/1 -> c/1
  c_to_ri/1 -> ri_to_c/1
  r/1 -> c_to_ri/1
  c_to_ri/2 -> ri_to_c/2

== system adc16_dbf_4fft/4fft5/mult_j ==
  a+jb : Inport
  Negate : xbsIndex_r4/Negate  precision=User Defined  arith_type="Signed  (2's comp)"  n_bits=18  bin_pt=17  quantization=Truncate  overflow=Wrap  en=off  latency=0  dbl_ovrd=off  block_type=negate
  c_to_ri : casper_library_misc/c_to_ri  n_bits=18  bin_pt=17
  ri_to_c : casper_library_misc/ri_to_c
  ja-b : Outport
  wires:
  Negate/1 -> ri_to_c/1
  c_to_ri/1 -> ri_to_c/2
  c_to_ri/2 -> Negate/1
  ri_to_c/1 -> ja-b/1
  a+jb/1 -> c_to_ri/1

== system adc16_dbf_4fft/4fft5/mult_jjj ==
  a+jb : Inport
  Negate : xbsIndex_r4/Negate  precision=User Defined  arith_type="Signed  (2's comp)"  n_bits=18  bin_pt=17  quantization=Truncate  overflow=Wrap  en=off  latency=0  dbl_ovrd=off  block_type=negate
  c_to_ri : casper_library_misc/c_to_ri  n_bits=18  bin_pt=17
  ri_to_c : casper_library_misc/ri_to_c
  b-ja : Outport
  wires:
  Negate/1 -> ri_to_c/2
  c_to_ri/1 -> Negate/1
  c_to_ri/2 -> ri_to_c/1
  a+jb/1 -> c_to_ri/1
  ri_to_c/1 -> b-ja/1

== system adc16_dbf_4fft/4fft5/pipeline ==
  d : Inport
  Register{0..3} (4 alike) : xbsIndex_r4/Register  init=0  rst=off  en=off  dbl_ovrd=off  block_type=register
      Register0 settings: block_version=11.4
      Register1 settings: block_version=11.4
  q : Outport
  wires:
  Register3/1 -> q/1
  d/1 -> Register0/1
  Register2/1 -> Register3/1
  Register1/1 -> Register2/1
  Register0/1 -> Register1/1

== system adc16_dbf_4fft/4fft5/pipeline1 ==
  d : Inport
  Register{0..3} (4 alike) : xbsIndex_r4/Register  init=0  rst=off  en=off  dbl_ovrd=off  block_type=register
      Register0 settings: block_version=11.4
      Register1 settings: block_version=11.4
  q : Outport
  wires:
  Register3/1 -> q/1
  d/1 -> Register0/1
  Register2/1 -> Register3/1
  Register1/1 -> Register2/1
  Register0/1 -> Register1/1

== system adc16_dbf_4fft/4fft5/real2complex ==
  r : Inport
  c_to_ri : casper_library_misc/c_to_ri  n_bits=18  bin_pt=17
  ri_to_c : casper_library_misc/ri_to_c
  c : Outport
  wires:
  ri_to_c/1 -> c/1
  c_to_ri/1 -> ri_to_c/1
  r/1 -> c_to_ri/1
  c_to_ri/2 -> ri_to_c/2

== system adc16_dbf_4fft/4fft5/real2complex1 ==
  r : Inport
  c_to_ri : casper_library_misc/c_to_ri  n_bits=18  bin_pt=17
  ri_to_c : casper_library_misc/ri_to_c
  c : Outport
  wires:
  c_to_ri/2 -> ri_to_c/2
  r/1 -> c_to_ri/1
  c_to_ri/1 -> ri_to_c/1
  ri_to_c/1 -> c/1

== system adc16_dbf_4fft/4fft5/real2complex2 ==
  r : Inport
  c_to_ri : casper_library_misc/c_to_ri  n_bits=18  bin_pt=17
  ri_to_c : casper_library_misc/ri_to_c
  c : Outport
  wires:
  ri_to_c/1 -> c/1
  c_to_ri/1 -> ri_to_c/1
  r/1 -> c_to_ri/1
  c_to_ri/2 -> ri_to_c/2

== system adc16_dbf_4fft/4fft5/real2complex3 ==
  r : Inport
  c_to_ri : casper_library_misc/c_to_ri  n_bits=18  bin_pt=17
  ri_to_c : casper_library_misc/ri_to_c
  c : Outport
  wires:
  c_to_ri/2 -> ri_to_c/2
  r/1 -> c_to_ri/1
  c_to_ri/1 -> ri_to_c/1
  ri_to_c/1 -> c/1

== system adc16_dbf_4fft/4fft6/mult_j ==
  a+jb : Inport
  Negate : xbsIndex_r4/Negate  precision=User Defined  arith_type="Signed  (2's comp)"  n_bits=18  bin_pt=17  quantization=Truncate  overflow=Wrap  en=off  latency=0  dbl_ovrd=off  block_type=negate
  c_to_ri : casper_library_misc/c_to_ri  n_bits=18  bin_pt=17
  ri_to_c : casper_library_misc/ri_to_c
  ja-b : Outport
  wires:
  a+jb/1 -> c_to_ri/1
  ri_to_c/1 -> ja-b/1
  c_to_ri/2 -> Negate/1
  c_to_ri/1 -> ri_to_c/2
  Negate/1 -> ri_to_c/1

== system adc16_dbf_4fft/4fft6/mult_jjj ==
  a+jb : Inport
  Negate : xbsIndex_r4/Negate  precision=User Defined  arith_type="Signed  (2's comp)"  n_bits=18  bin_pt=17  quantization=Truncate  overflow=Wrap  en=off  latency=0  dbl_ovrd=off  block_type=negate
  c_to_ri : casper_library_misc/c_to_ri  n_bits=18  bin_pt=17
  ri_to_c : casper_library_misc/ri_to_c
  b-ja : Outport
  wires:
  ri_to_c/1 -> b-ja/1
  a+jb/1 -> c_to_ri/1
  c_to_ri/2 -> ri_to_c/1
  c_to_ri/1 -> Negate/1
  Negate/1 -> ri_to_c/2

== system adc16_dbf_4fft/4fft6/pipeline ==
  d : Inport
  Register{0..3} (4 alike) : xbsIndex_r4/Register  init=0  rst=off  en=off  dbl_ovrd=off  block_type=register
      Register0 settings: block_version=11.4
      Register1 settings: block_version=11.4
  q : Outport
  wires:
  Register0/1 -> Register1/1
  Register1/1 -> Register2/1
  Register2/1 -> Register3/1
  d/1 -> Register0/1
  Register3/1 -> q/1

== system adc16_dbf_4fft/4fft6/pipeline1 ==
  d : Inport
  Register{0..3} (4 alike) : xbsIndex_r4/Register  init=0  rst=off  en=off  dbl_ovrd=off  block_type=register
      Register0 settings: block_version=11.4
      Register1 settings: block_version=11.4
  q : Outport
  wires:
  Register0/1 -> Register1/1
  Register1/1 -> Register2/1
  Register2/1 -> Register3/1
  d/1 -> Register0/1
  Register3/1 -> q/1

== system adc16_dbf_4fft/4fft6/real2complex ==
  r : Inport
  c_to_ri : casper_library_misc/c_to_ri  n_bits=18  bin_pt=17
  ri_to_c : casper_library_misc/ri_to_c
  c : Outport
  wires:
  c_to_ri/2 -> ri_to_c/2
  r/1 -> c_to_ri/1
  c_to_ri/1 -> ri_to_c/1
  ri_to_c/1 -> c/1

== system adc16_dbf_4fft/4fft6/real2complex1 ==
  r : Inport
  c_to_ri : casper_library_misc/c_to_ri  n_bits=18  bin_pt=17
  ri_to_c : casper_library_misc/ri_to_c
  c : Outport
  wires:
  ri_to_c/1 -> c/1
  c_to_ri/1 -> ri_to_c/1
  r/1 -> c_to_ri/1
  c_to_ri/2 -> ri_to_c/2

== system adc16_dbf_4fft/4fft6/real2complex2 ==
  r : Inport
  c_to_ri : casper_library_misc/c_to_ri  n_bits=18  bin_pt=17
  ri_to_c : casper_library_misc/ri_to_c
  c : Outport
  wires:
  c_to_ri/2 -> ri_to_c/2
  r/1 -> c_to_ri/1
  c_to_ri/1 -> ri_to_c/1
  ri_to_c/1 -> c/1

== system adc16_dbf_4fft/4fft6/real2complex3 ==
  r : Inport
  c_to_ri : casper_library_misc/c_to_ri  n_bits=18  bin_pt=17
  ri_to_c : casper_library_misc/ri_to_c
  c : Outport
  wires:
  ri_to_c/1 -> c/1
  c_to_ri/1 -> ri_to_c/1
  r/1 -> c_to_ri/1
  c_to_ri/2 -> ri_to_c/2

== system adc16_dbf_4fft/4fft7/mult_j ==
  a+jb : Inport
  Negate : xbsIndex_r4/Negate  precision=User Defined  arith_type="Signed  (2's comp)"  n_bits=18  bin_pt=17  quantization=Truncate  overflow=Wrap  en=off  latency=0  dbl_ovrd=off  block_type=negate
  c_to_ri : casper_library_misc/c_to_ri  n_bits=18  bin_pt=17
  ri_to_c : casper_library_misc/ri_to_c
  ja-b : Outport
  wires:
  Negate/1 -> ri_to_c/1
  c_to_ri/1 -> ri_to_c/2
  c_to_ri/2 -> Negate/1
  ri_to_c/1 -> ja-b/1
  a+jb/1 -> c_to_ri/1

== system adc16_dbf_4fft/4fft7/mult_jjj ==
  a+jb : Inport
  Negate : xbsIndex_r4/Negate  precision=User Defined  arith_type="Signed  (2's comp)"  n_bits=18  bin_pt=17  quantization=Truncate  overflow=Wrap  en=off  latency=0  dbl_ovrd=off  block_type=negate
  c_to_ri : casper_library_misc/c_to_ri  n_bits=18  bin_pt=17
  ri_to_c : casper_library_misc/ri_to_c
  b-ja : Outport
  wires:
  Negate/1 -> ri_to_c/2
  c_to_ri/1 -> Negate/1
  c_to_ri/2 -> ri_to_c/1
  a+jb/1 -> c_to_ri/1
  ri_to_c/1 -> b-ja/1

== system adc16_dbf_4fft/4fft7/pipeline ==
  d : Inport
  Register{0..3} (4 alike) : xbsIndex_r4/Register  init=0  rst=off  en=off  dbl_ovrd=off  block_type=register
      Register0 settings: block_version=11.4
      Register1 settings: block_version=11.4
  q : Outport
  wires:
  Register3/1 -> q/1
  d/1 -> Register0/1
  Register2/1 -> Register3/1
  Register1/1 -> Register2/1
  Register0/1 -> Register1/1

== system adc16_dbf_4fft/4fft7/pipeline1 ==
  d : Inport
  Register{0..3} (4 alike) : xbsIndex_r4/Register  init=0  rst=off  en=off  dbl_ovrd=off  block_type=register
      Register0 settings: block_version=11.4
      Register1 settings: block_version=11.4
  q : Outport
  wires:
  Register3/1 -> q/1
  d/1 -> Register0/1
  Register2/1 -> Register3/1
  Register1/1 -> Register2/1
  Register0/1 -> Register1/1

== system adc16_dbf_4fft/4fft7/real2complex ==
  r : Inport
  c_to_ri : casper_library_misc/c_to_ri  n_bits=18  bin_pt=17
  ri_to_c : casper_library_misc/ri_to_c
  c : Outport
  wires:
  ri_to_c/1 -> c/1
  c_to_ri/1 -> ri_to_c/1
  r/1 -> c_to_ri/1
  c_to_ri/2 -> ri_to_c/2

== system adc16_dbf_4fft/4fft7/real2complex1 ==
  r : Inport
  c_to_ri : casper_library_misc/c_to_ri  n_bits=18  bin_pt=17
  ri_to_c : casper_library_misc/ri_to_c
  c : Outport
  wires:
  c_to_ri/2 -> ri_to_c/2
  r/1 -> c_to_ri/1
  c_to_ri/1 -> ri_to_c/1
  ri_to_c/1 -> c/1

== system adc16_dbf_4fft/4fft7/real2complex2 ==
  r : Inport
  c_to_ri : casper_library_misc/c_to_ri  n_bits=18  bin_pt=17
  ri_to_c : casper_library_misc/ri_to_c
  c : Outport
  wires:
  ri_to_c/1 -> c/1
  c_to_ri/1 -> ri_to_c/1
  r/1 -> c_to_ri/1
  c_to_ri/2 -> ri_to_c/2

== system adc16_dbf_4fft/4fft7/real2complex3 ==
  r : Inport
  c_to_ri : casper_library_misc/c_to_ri  n_bits=18  bin_pt=17
  ri_to_c : casper_library_misc/ri_to_c
  c : Outport
  wires:
  c_to_ri/2 -> ri_to_c/2
  r/1 -> c_to_ri/1
  c_to_ri/1 -> ri_to_c/1
  ri_to_c/1 -> c/1

== system adc16_dbf_4fft/bus_power2scope/gateway21 ==
  data[4] : Inport
  Bus Creator : BusCreator
  Bus Selector : BusSelector  OutputSignals=signal1,signal2,signal3,signal4
  Gateway Out{,1..3} (4 alike) : xbsIndex_r4/Gateway Out  inherit_from_input=off  hdl_port=on  timing_constraint=None  locs_specified=off  LOCs={}  UseAsDAC=off  DACChannel='1'  block_type=gatewayout
  to_scope : Outport
  wires:
  data[4]/1 -> Bus Selector/1
  Bus Selector/4 -> Gateway Out3/1  "<signal4>"
  Bus Selector/2 -> Gateway Out1/1  "<signal2>"
  Bus Selector/1 -> Gateway Out/1  "<signal1>"
  Bus Selector/3 -> Gateway Out2/1  "<signal3>"
  Bus Creator/1 -> to_scope/1
  Gateway Out/1 -> Bus Creator/1
  Gateway Out1/1 -> Bus Creator/2
  Gateway Out2/1 -> Bus Creator/3
  Gateway Out3/1 -> Bus Creator/4

== system adc16_dbf_4fft/bus_power2scope1/gateway21 ==
  data[4] : Inport
  Bus Creator : BusCreator
  Bus Selector : BusSelector  OutputSignals=signal1,signal2,signal3,signal4
  Gateway Out{,1..3} (4 alike) : xbsIndex_r4/Gateway Out  inherit_from_input=off  hdl_port=on  timing_constraint=None  locs_specified=off  LOCs={}  UseAsDAC=off  DACChannel='1'  block_type=gatewayout
  to_scope : Outport
  wires:
  Gateway Out3/1 -> Bus Creator/4
  Gateway Out2/1 -> Bus Creator/3
  Gateway Out1/1 -> Bus Creator/2
  Gateway Out/1 -> Bus Creator/1
  Bus Creator/1 -> to_scope/1
  Bus Selector/3 -> Gateway Out2/1  "<signal3>"
  Bus Selector/1 -> Gateway Out/1  "<signal1>"
  Bus Selector/2 -> Gateway Out1/1  "<signal2>"
  Bus Selector/4 -> Gateway Out3/1  "<signal4>"
  data[4]/1 -> Bus Selector/1

== system adc16_dbf_4fft/bus_power2scope2/gateway21 ==
  data[4] : Inport
  Bus Creator : BusCreator
  Bus Selector : BusSelector  OutputSignals=signal1,signal2,signal3,signal4
  Gateway Out{,1..3} (4 alike) : xbsIndex_r4/Gateway Out  inherit_from_input=off  hdl_port=on  timing_constraint=None  locs_specified=off  LOCs={}  UseAsDAC=off  DACChannel='1'  block_type=gatewayout
  to_scope : Outport
  wires:
  data[4]/1 -> Bus Selector/1
  Bus Selector/4 -> Gateway Out3/1  "<signal4>"
  Bus Selector/2 -> Gateway Out1/1  "<signal2>"
  Bus Selector/1 -> Gateway Out/1  "<signal1>"
  Bus Selector/3 -> Gateway Out2/1  "<signal3>"
  Bus Creator/1 -> to_scope/1
  Gateway Out/1 -> Bus Creator/1
  Gateway Out1/1 -> Bus Creator/2
  Gateway Out2/1 -> Bus Creator/3
  Gateway Out3/1 -> Bus Creator/4

== system adc16_dbf_4fft/bus_power2scope3/gateway21 ==
  data[4] : Inport
  Bus Creator : BusCreator
  Bus Selector : BusSelector  OutputSignals=signal1,signal2,signal3,signal4
  Gateway Out{,1..3} (4 alike) : xbsIndex_r4/Gateway Out  inherit_from_input=off  hdl_port=on  timing_constraint=None  locs_specified=off  LOCs={}  UseAsDAC=off  DACChannel='1'  block_type=gatewayout
  to_scope : Outport
  wires:
  Gateway Out3/1 -> Bus Creator/4
  Gateway Out2/1 -> Bus Creator/3
  Gateway Out1/1 -> Bus Creator/2
  Gateway Out/1 -> Bus Creator/1
  Bus Creator/1 -> to_scope/1
  Bus Selector/3 -> Gateway Out2/1  "<signal3>"
  Bus Selector/1 -> Gateway Out/1  "<signal1>"
  Bus Selector/2 -> Gateway Out1/1  "<signal2>"
  Bus Selector/4 -> Gateway Out3/1  "<signal4>"
  data[4]/1 -> Bus Selector/1

== system adc16_dbf_4fft/hold_data/power_integrator ==
  data : Inport
  en : Inport  Port=2
  Register : xbsIndex_r4/Register  init=0  rst=off  en=on  dbl_ovrd=off  block_type=register
  pow : Outport
  wires:
  data/1 -> Register/1
  Register/1 -> pow/1
  en/1 -> Register/2

== system adc16_dbf_4fft/hold_data/power_integrator1 ==
  data : Inport
  en : Inport  Port=2
  Register : xbsIndex_r4/Register  init=0  rst=off  en=on  dbl_ovrd=off  block_type=register
  pow : Outport
  wires:
  en/1 -> Register/2
  Register/1 -> pow/1
  data/1 -> Register/1

== system adc16_dbf_4fft/hold_data/power_integrator10 ==
  data : Inport
  en : Inport  Port=2
  Register : xbsIndex_r4/Register  init=0  rst=off  en=on  dbl_ovrd=off  block_type=register
  pow : Outport
  wires:
  en/1 -> Register/2
  Register/1 -> pow/1
  data/1 -> Register/1

== system adc16_dbf_4fft/hold_data/power_integrator11 ==
  data : Inport
  en : Inport  Port=2
  Register : xbsIndex_r4/Register  init=0  rst=off  en=on  dbl_ovrd=off  block_type=register
  pow : Outport
  wires:
  data/1 -> Register/1
  Register/1 -> pow/1
  en/1 -> Register/2

== system adc16_dbf_4fft/hold_data/power_integrator12 ==
  data : Inport
  en : Inport  Port=2
  Register : xbsIndex_r4/Register  init=0  rst=off  en=on  dbl_ovrd=off  block_type=register
  pow : Outport
  wires:
  en/1 -> Register/2
  Register/1 -> pow/1
  data/1 -> Register/1

== system adc16_dbf_4fft/hold_data/power_integrator13 ==
  data : Inport
  en : Inport  Port=2
  Register : xbsIndex_r4/Register  init=0  rst=off  en=on  dbl_ovrd=off  block_type=register
  pow : Outport
  wires:
  data/1 -> Register/1
  Register/1 -> pow/1
  en/1 -> Register/2

== system adc16_dbf_4fft/hold_data/power_integrator14 ==
  data : Inport
  en : Inport  Port=2
  Register : xbsIndex_r4/Register  init=0  rst=off  en=on  dbl_ovrd=off  block_type=register
  pow : Outport
  wires:
  en/1 -> Register/2
  Register/1 -> pow/1
  data/1 -> Register/1

== system adc16_dbf_4fft/hold_data/power_integrator15 ==
  data : Inport
  en : Inport  Port=2
  Register : xbsIndex_r4/Register  init=0  rst=off  en=on  dbl_ovrd=off  block_type=register
  pow : Outport
  wires:
  data/1 -> Register/1
  Register/1 -> pow/1
  en/1 -> Register/2

== system adc16_dbf_4fft/hold_data/power_integrator2 ==
  data : Inport
  en : Inport  Port=2
  Register : xbsIndex_r4/Register  init=0  rst=off  en=on  dbl_ovrd=off  block_type=register
  pow : Outport
  wires:
  data/1 -> Register/1
  Register/1 -> pow/1
  en/1 -> Register/2

== system adc16_dbf_4fft/hold_data/power_integrator3 ==
  data : Inport
  en : Inport  Port=2
  Register : xbsIndex_r4/Register  init=0  rst=off  en=on  dbl_ovrd=off  block_type=register
  pow : Outport
  wires:
  en/1 -> Register/2
  Register/1 -> pow/1
  data/1 -> Register/1

== system adc16_dbf_4fft/hold_data/power_integrator4 ==
  data : Inport
  en : Inport  Port=2
  Register : xbsIndex_r4/Register  init=0  rst=off  en=on  dbl_ovrd=off  block_type=register
  pow : Outport
  wires:
  data/1 -> Register/1
  Register/1 -> pow/1
  en/1 -> Register/2

== system adc16_dbf_4fft/hold_data/power_integrator5 ==
  data : Inport
  en : Inport  Port=2
  Register : xbsIndex_r4/Register  init=0  rst=off  en=on  dbl_ovrd=off  block_type=register
  pow : Outport
  wires:
  en/1 -> Register/2
  Register/1 -> pow/1
  data/1 -> Register/1

== system adc16_dbf_4fft/hold_data/power_integrator6 ==
  data : Inport
  en : Inport  Port=2
  Register : xbsIndex_r4/Register  init=0  rst=off  en=on  dbl_ovrd=off  block_type=register
  pow : Outport
  wires:
  data/1 -> Register/1
  Register/1 -> pow/1
  en/1 -> Register/2

== system adc16_dbf_4fft/hold_data/power_integrator7 ==
  data : Inport
  en : Inport  Port=2
  Register : xbsIndex_r4/Register  init=0  rst=off  en=on  dbl_ovrd=off  block_type=register
  pow : Outport
  wires:
  en/1 -> Register/2
  Register/1 -> pow/1
  data/1 -> Register/1

== system adc16_dbf_4fft/hold_data/power_integrator8 ==
  data : Inport
  en : Inport  Port=2
  Register : xbsIndex_r4/Register  init=0  rst=off  en=on  dbl_ovrd=off  block_type=register
  pow : Outport
  wires:
  en/1 -> Register/2
  Register/1 -> pow/1
  data/1 -> Register/1

== system adc16_dbf_4fft/hold_data/power_integrator9 ==
  data : Inport
  en : Inport  Port=2
  Register : xbsIndex_r4/Register  init=0  rst=off  en=on  dbl_ovrd=off  block_type=register
  pow : Outport
  wires:
  data/1 -> Register/1
  Register/1 -> pow/1
  en/1 -> Register/2

== system adc16_dbf_4fft/hold_data1/power_integrator ==
  data : Inport
  en : Inport  Port=2
  Register : xbsIndex_r4/Register  init=0  rst=off  en=on  dbl_ovrd=off  block_type=register
  pow : Outport
  wires:
  en/1 -> Register/2
  Register/1 -> pow/1
  data/1 -> Register/1

== system adc16_dbf_4fft/hold_data1/power_integrator1 ==
  data : Inport
  en : Inport  Port=2
  Register : xbsIndex_r4/Register  init=0  rst=off  en=on  dbl_ovrd=off  block_type=register
  pow : Outport
  wires:
  data/1 -> Register/1
  Register/1 -> pow/1
  en/1 -> Register/2

== system adc16_dbf_4fft/hold_data1/power_integrator10 ==
  data : Inport
  en : Inport  Port=2
  Register : xbsIndex_r4/Register  init=0  rst=off  en=on  dbl_ovrd=off  block_type=register
  pow : Outport
  wires:
  data/1 -> Register/1
  Register/1 -> pow/1
  en/1 -> Register/2

== system adc16_dbf_4fft/hold_data1/power_integrator11 ==
  data : Inport
  en : Inport  Port=2
  Register : xbsIndex_r4/Register  init=0  rst=off  en=on  dbl_ovrd=off  block_type=register
  pow : Outport
  wires:
  en/1 -> Register/2
  Register/1 -> pow/1
  data/1 -> Register/1

== system adc16_dbf_4fft/hold_data1/power_integrator12 ==
  data : Inport
  en : Inport  Port=2
  Register : xbsIndex_r4/Register  init=0  rst=off  en=on  dbl_ovrd=off  block_type=register
  pow : Outport
  wires:
  data/1 -> Register/1
  Register/1 -> pow/1
  en/1 -> Register/2

== system adc16_dbf_4fft/hold_data1/power_integrator13 ==
  data : Inport
  en : Inport  Port=2
  Register : xbsIndex_r4/Register  init=0  rst=off  en=on  dbl_ovrd=off  block_type=register
  pow : Outport
  wires:
  en/1 -> Register/2
  Register/1 -> pow/1
  data/1 -> Register/1
